simulink model "interpolation_nD_TestGen70"  (R2017b)
settings: Solver=FixedStepDiscrete  StartTime=0.0  StopTime=10.0  RelTol=1e-3
PreLoadFcn:
  |  LUTObj = Simulink.LookupTable;
  |  LUTObj.Table.Value = reshape(repmat([4 5 6 7 8;16 19 20 21 22;10 18 23 24 25],2,2),[2,5,3,2]);
  |  LUTObj.Table.DataType = 'auto';
  |  LUTObj.StructTypeInfo.Name = 'myLUTStruct';
  |  LUTObj.BreakpointsSpecification = 'Reference';
  |  LUTObj.Breakpoints{1} = 'myBpSet1';
  | myBpSet1 = Simulink.Breakpoint;
  | myBpSet1.Breakpoints.Value = [1 2];
  |  LUTObj.Breakpoints{2} = 'myBpSet2';
  | myBpSet2 = Simulink.Breakpoint;
  | myBpSet2.Breakpoints.Value = [1 2 3 4 5];
  |  LUTObj.Breakpoints{3} = 'myBpSet3';
  | myBpSet3 = Simulink.Breakpoint;
  | myBpSet3.Breakpoints.Value = [1 2 3];
  |  LUTObj.Breakpoints{4} = 'myBpSet4';
  | myBpSet4 = Simulink.Breakpoint;
  | myBpSet4.Breakpoints.Value = [1 2];
settings Model: Creator=ktrinh  LastModifiedBy=ktrinh
settings DebuggingCC: ParameterOverflowMsg=none

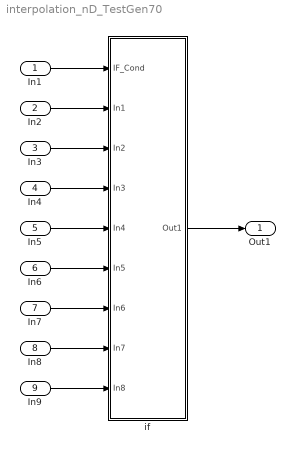
== system interpolation_nD_TestGen70 ==
  In1 : Inport
  In2 : Inport  Port=2
  In3 : Inport  Port=3
  In4 : Inport  Port=4
  In5 : Inport  Port=5
  In6 : Inport  Port=6
  In7 : Inport  Port=7
  In8 : Inport  Port=8
  In9 : Inport  Port=9
  if : Subsystem  AncestorBlock=Block_TestLib/if
  Out1 : Outport
  wires:
  In1/1 -> if/1(IF_Cond)
  In2/1 -> if/2(In1)
  In3/1 -> if/3(In2)
  In4/1 -> if/4(In3)
  In5/1 -> if/5(In4)
  In6/1 -> if/6(In5)
  In7/1 -> if/7(In6)
  In8/1 -> if/8(In7)
  In9/1 -> if/9(In8)
  if/1(Out1) -> Out1/1

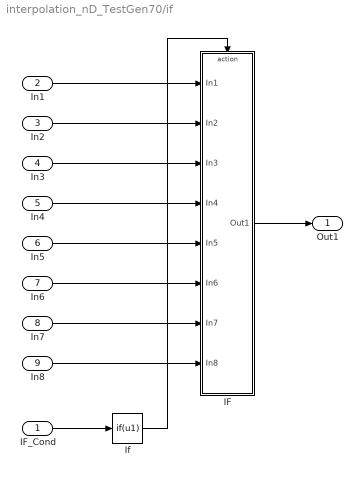
== system interpolation_nD_TestGen70/if ==
  IF_Cond : Inport  OutDataTypeStr=boolean
  In1 : Inport  Port=2
  In2 : Inport  Port=3
  In3 : Inport  Port=4
  In4 : Inport  Port=5
  In5 : Inport  Port=6
  In6 : Inport  Port=7
  In7 : Inport  Port=8
  In8 : Inport  Port=9
  IF : Subsystem  TreatAsAtomicUnit=on
  If : If  IfExpression=u1  ShowElse=off
  Out1 : Outport
  wires:
  If/1 -> IF/Action
  In1/1 -> IF/1(In1)
  In2/1 -> IF/2(In2)
  In3/1 -> IF/3(In3)
  In4/1 -> IF/4(In4)
  In5/1 -> IF/5(In5)
  In6/1 -> IF/6(In6)
  In7/1 -> IF/7(In7)
  In8/1 -> IF/8(In8)
  IF_Cond/1 -> If/1
  IF/1(Out1) -> Out1/1

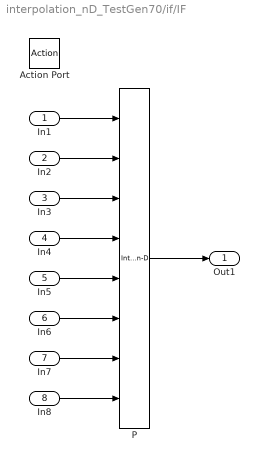
== system interpolation_nD_TestGen70/if/IF ==
  In1 : Inport  OutMin=0  OutMax=2  PortDimensions=1
  In2 : Inport  Port=2  OutMin=-0.5  OutMax=1.5
  In3 : Inport  Port=3  OutMin=0  OutMax=5
  In4 : Inport  Port=4  OutMin=-0.5  OutMax=1.5
  In5 : Inport  Port=5  OutMin=0  OutMax=3
  In6 : Inport  Port=6  OutMin=-0.5  OutMax=1.5
  In7 : Inport  Port=7  OutMin=0  OutMax=2
  In8 : Inport  Port=8  OutMin=-0.5  OutMax=1.5
  Action Port : ActionPort  ActionType=then
  P : Interpolation_n-D  NumberOfTableDimensions=4  Table=reshape(repmat([4 5 6 7 8;16 19 20 21 22;10 18 23 24 25],2,2),[2,5,3,2])  TableSpecification=Lookup table object  LookupTableObject=LUTObj  InterpMethod=Nearest  OutDataTypeStr=Inherit: Inherit via back propagation  InternalRulePriority=Speed  RndMeth=Ceiling
      settings: InputPortMap=u0,u1,u2,u3,u4,u5,u6,u7
  Out1 : Outport
  wires:
  In1/1 -> P/1
  In2/1 -> P/2
  In3/1 -> P/3
  In4/1 -> P/4
  In5/1 -> P/5
  In6/1 -> P/6
  In7/1 -> P/7
  In8/1 -> P/8
  P/1 -> Out1/1
